simulink model "sampleModel1491"  (R2023a)
settings: Solver=VariableStepAuto  StartTime=0.0  StopTime=10.0  RelTol=1e-3
libraries: simulink x3, hdlsllib x2
settings Model: Creator=user1  LastModifiedBy=user1

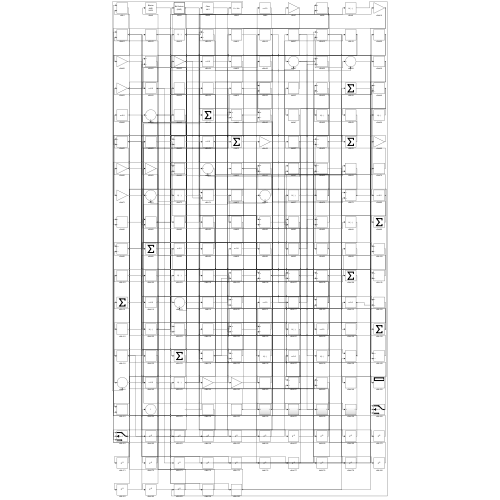
[thumbnail: Simulink's stored preview of the top-level diagram]
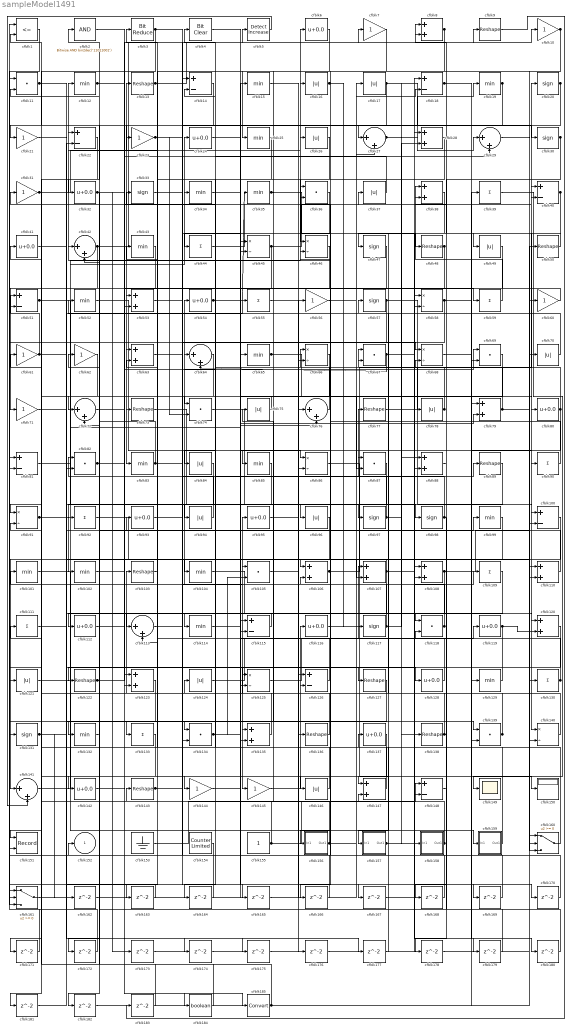
== system sampleModel1491 ==
  cfblk1 : RelationalOperator  Operator=<=  OutDataTypeStr=boolean  InputSameDT=off
  cfblk{7,10,21,23,31,56,60..62,71,144..145} (12 alike) : Gain
  cfblk{14,18,22,40,51,81,100,115,126,148} (10 alike) : Sum  Inputs=+-
  cfblk{12,15,19,25,34..35,43,52,65,83,85,99,101..102,104,114,129,132} (18 alike) : MinMax
  cfblk{9,13,48,50,73,77,89,103,122,127,136,138,143} (13 alike) : Reshape
  cfblk{11,36,67,69,74,82,87,105,118,134,139} (11 alike) : DotProduct  OutDataTypeStr=Inherit: Inherit via internal rule
  cfblk{8,28,38,53,63,79,88,106..108,110,120,123,135,147} (15 alike) : Sum
  cfblk{39,44,55,59,90,92,109,111,130,133} (10 alike) : Sum  Inputs=+
  cfblk{6,24,32,41,54,80,93,95,112,116,119,128,137,142} (14 alike) : Bias  Bias=0.0  SaturateOnIntegerOverflow=off
  cfblk{27,29,42,64,72,76,113,141} (8 alike) : Sum  Inputs=|++
  cfblk{20,30,33,47,57,97..98,117,131} (9 alike) : Signum
  cfblk{16..17,26,37,49,70,75,78,84,94,96,121,124,146} (14 alike) : Abs  SaturateOnIntegerOverflow=off
  cfblk{45..46,58,66,68,86,91,125,140} (9 alike) : Product  Inputs=*/  RndMeth=Zero  SaturateOnIntegerOverflow=on
  cfblk149 : Scope
  cfblk150 : Display
  cfblk151 : Record  FileSettingsInternal="{\"entries\":[{\"content\":{\"excelSettings\":{\"content\":{},\"type\":\"Streamout.ExcelSettings\"}},\"type\":\"Streamout.FileSettingStorage\",\"uuid\":\"\"}],\"packageUris\":[\"http:\\/\\/schema.mathworks.com\\/mf0\\/streamout_blocks\\/R2020a\"],\"version\":\"1.0\"}"  Layout=[1 1]  SignalsInternal="{\"entries\":[{\"content\":{\"signals\":[{\"content\":{\"blockPath\":[],\"dimensions\":[1],\"domain\":\"\",\"lineColor\":\"#a2142f\",\"plots\":[1],\"port\":1,\"signalID\":1220,\"signalName\":\"XY Graph:1\"},\"type\":\"RecordBlkView.Signal\",\"uuid\":\"\"},{\"content\":{\"blockPath\":[],\"dimensions\":[1],\"domain\":\"\",\"lineColor\":\"#139fff\",\"plots\":[1],\"port\":2,\"signalID\":1223,\"signalName\":\"XY Graph:2\"},\"type\":\"RecordBlkView.Signal\",\"uuid\":\"\"}]},\"type\":\"RecordBlkView.InputSignals\",\"uuid\":\"\"}],\"packageUris\":[\"http:\\/\\/schema.mathworks.com\\/mf0\\/streamout_blocks\\/R2020a\"],\"version\":\"1.0\"}"  VisualizationBindings="{\"xyplotplugin\":{\"info\":[{\"series\":[{\"bindingParametersList\":[{\"parameter\":\"X-Axis\",\"signalID\":1220,\"signalName\":\"XY Graph:1\"},{\"parameter\":\"Y-Axis\",\"signalID\":1223,\"signalName\":\"XY Graph:2\"}],\"seriesID\":24875}],\"subplotID\":1}]}}"  CompatibilityTag=XY  st=-1
  cfblk153 : Ground
  cfblk154 : hdlsllib/Sources/Counter Limited  uplimit=7  tsamp=-1
  cfblk155 : Constant  SampleTime=-1
  cfblk156 : Subsystem
      settings: LibrarySourceBlock=|
      | hdlsllib/Ports &
      | Subsystems/Subsystem
  cfblk157 : Subsystem
      settings: LibrarySourceBlock=|
      | hdlsllib/Ports &
      | Subsystems/Subsystem
  cfblk158 : Subsystem
      settings: LibrarySourceBlock=|
      | hdlsllib/Ports &
      | Subsystems/Subsystem
  cfblk159 : Subsystem
      settings: LibrarySourceBlock=|
      | hdlsllib/Ports &
      | Subsystems/Subsystem
  cfblk160 : Switch  SaturateOnIntegerOverflow=off  InputSameDT=off
  cfblk161 : Switch  SaturateOnIntegerOverflow=off  InputSameDT=off
  cfblk{162..183} (22 alike) : Delay  SampleTime=1
  cfblk184 : DataTypeConversion  OutDataTypeStr=boolean  SaturateOnIntegerOverflow=off  RndMeth=Floor
  cfblk185 : DataTypeConversion  SaturateOnIntegerOverflow=off  RndMeth=Floor
  cfblk2 : simulink/Logic and Bit Operations/Bitwise Operator  logicop=AND  UseBitMask=on  BitMask=bin2dec('11011001')  BitMaskRealWorld=Stored Integer
      settings: LibrarySourceBlock=|
      | hdlsllib/Logic and Bit
      | Operations/Bitwise
      | Operator
  cfblk3 : hdlsllib/Logic and Bit Operations/Bit Reduce  mode=AND
  cfblk4 : simulink/Logic and Bit Operations/Bit Clear  iBit=0
      settings: LibrarySourceBlock=|
      | hdlsllib/Logic and Bit
      | Operations/Bit Clear
  cfblk5 : simulink/Logic and Bit Operations/Detect Increase  vinit=0.0  OutDataTypeStr=boolean
      settings: LibrarySourceBlock=|
      | hdlsllib/Logic and Bit
      | Operations/Detect
      | Increase
  cfblk152 : Outport  VectorParamsAs1DForOutWhenUnconnected=off
  wires:
  cfblk42/1 -> cfblk10/1, cfblk127/1, cfblk82/2
  cfblk3/1 -> cfblk21/1, cfblk169/1
  cfblk126/1 -> cfblk12/1
  cfblk155/1 -> cfblk148/1, cfblk143/1
  cfblk90/1 -> cfblk42/1
  cfblk121/1 -> cfblk6/1
  cfblk128/1 -> cfblk22/1
  cfblk120/1 -> cfblk103/1
  cfblk39/1 -> cfblk149/1
  cfblk135/1 -> cfblk95/1
  cfblk67/1 -> cfblk64/2, cfblk179/1
  cfblk119/1 -> cfblk145/1, cfblk120/2
  cfblk12/1 -> cfblk59/1, cfblk184/1
  cfblk123/1 -> cfblk141/1
  cfblk127/1 -> cfblk133/1
  cfblk102/1 -> cfblk69/1
  cfblk14/1 -> cfblk83/1
  cfblk40/1 -> cfblk140/1, cfblk47/1
  cfblk144/1 -> cfblk119/1
  cfblk10/1 -> cfblk113/1, cfblk160/3
  cfblk117/1 -> cfblk54/1, cfblk88/1
  cfblk101/1 -> cfblk159/1(In1)
  cfblk54/1 -> cfblk35/1, cfblk84/1
  cfblk112/1 -> cfblk99/1
  cfblk8/1 -> cfblk25/1, cfblk36/1
  cfblk62/1 -> cfblk91/1
  cfblk5/1 -> cfblk141/2
  cfblk141/1 -> cfblk24/1
  cfblk76/1 -> cfblk31/1
  cfblk23/1 -> cfblk27/1, cfblk74/2
  cfblk78/1 -> cfblk67/1, cfblk67/2
  cfblk31/1 -> cfblk13/1, cfblk110/2
  cfblk59/1 -> cfblk38/1
  cfblk87/1 -> cfblk94/1
  cfblk57/1 -> cfblk100/1, cfblk151/2
  cfblk50/1 -> cfblk49/1
  cfblk48/1 -> cfblk147/1, cfblk88/2
  cfblk7/1 -> cfblk113/2
  cfblk51/1 -> cfblk96/1, cfblk175/1
  cfblk86/1 -> cfblk150/1
  cfblk73/1 -> cfblk115/1
  cfblk133/1 -> cfblk151/1
  cfblk116/1 -> cfblk148/2
  cfblk13/1 -> cfblk5/1, cfblk45/2
  cfblk60/1 -> cfblk53/1
  cfblk27/1 -> cfblk19/1, cfblk29/1, cfblk158/1(In1)
  cfblk49/1 -> cfblk71/1
  cfblk92/1 -> cfblk140/2
  cfblk29/1 -> cfblk110/1
  cfblk145/1 -> cfblk116/1
  cfblk160/1 -> cfblk61/1
  cfblk72/1 -> cfblk123/1
  cfblk147/1 -> cfblk34/1
  cfblk68/1 -> cfblk129/1
  cfblk66/1 -> cfblk144/1
  cfblk85/1 -> cfblk114/1
  cfblk53/1 -> cfblk68/1
  cfblk115/1 -> cfblk112/1
  cfblk139/1 -> cfblk57/1, cfblk124/1
  cfblk100/1 -> cfblk131/1
  cfblk106/1 -> cfblk20/1, cfblk18/2
  cfblk97/1 -> cfblk77/1, cfblk28/2
  cfblk80/1 -> cfblk52/1, cfblk135/2
  cfblk52/1 -> cfblk136/1
  cfblk161/1 -> cfblk17/1
  cfblk19/1 -> cfblk63/1, cfblk53/2
  cfblk91/1 -> cfblk15/1, cfblk97/1
  cfblk75/1 -> cfblk72/1
  cfblk4/1 -> cfblk80/1
  cfblk124/1 -> cfblk56/1
  cfblk36/1 -> cfblk44/1
  cfblk110/1 -> cfblk72/2
  cfblk159/1(Out1) -> cfblk64/1
  cfblk44/1 -> cfblk16/1
  cfblk96/1 -> cfblk142/1
  cfblk58/1 -> cfblk106/1, cfblk40/2
  cfblk125/1 -> cfblk69/2
  cfblk98/1 -> cfblk4/1, cfblk178/1
  cfblk93/1 -> cfblk128/1
  cfblk79/1 -> cfblk60/1, cfblk46/2
  cfblk65/1 -> cfblk126/1, cfblk87/2
  cfblk16/1 -> cfblk146/1, cfblk117/1
  cfblk45/1 -> cfblk37/1, cfblk51/2
  cfblk136/1 -> cfblk125/1
  cfblk2/1 -> cfblk185/1
  cfblk108/1 -> cfblk50/1, cfblk156/1(In1)
  cfblk63/1 -> cfblk7/1
  cfblk88/1 -> cfblk38/2
  cfblk129/1 -> cfblk122/1
  cfblk61/1 -> cfblk51/1, cfblk55/1
  cfblk77/1 -> cfblk39/1
  cfblk130/1 -> cfblk106/2, cfblk107/1
  cfblk74/1 -> cfblk98/1
  cfblk22/1 -> cfblk121/1
  cfblk114/1 -> cfblk79/2
  cfblk118/1 -> cfblk101/1, cfblk43/1
  cfblk20/1 -> cfblk32/1, cfblk66/2
  cfblk82/1 -> cfblk40/1, cfblk107/2
  cfblk21/1 -> cfblk134/1
  cfblk15/1 -> cfblk30/1
  cfblk28/1 -> cfblk46/1
  cfblk157/1(Out1) -> cfblk137/1, cfblk109/1
  cfblk17/1 -> cfblk81/2, cfblk130/1, cfblk138/1
  cfblk154/1 -> cfblk152/1
  cfblk107/1 -> cfblk78/1, cfblk104/1, cfblk115/2
  cfblk56/1 -> cfblk27/2
  cfblk84/1 -> cfblk134/2
  cfblk18/1 -> cfblk90/1, cfblk180/1
  cfblk26/1 -> cfblk73/1
  cfblk131/1 -> cfblk93/1, cfblk162/1
  cfblk105/1 -> cfblk89/1
  cfblk122/1 -> cfblk26/1, cfblk8/2
  cfblk30/1 -> cfblk48/1, cfblk160/2
  cfblk71/1 -> cfblk125/2
  cfblk89/1 -> cfblk102/1
  cfblk156/1(Out1) -> cfblk41/1, cfblk66/1, cfblk118/2
  cfblk104/1 -> cfblk118/1
  cfblk134/1 -> cfblk105/2, cfblk170/1
  cfblk24/1 -> cfblk86/1
  cfblk35/1 -> cfblk135/1, cfblk58/2
  cfblk95/1 -> cfblk108/2
  cfblk103/1 -> cfblk3/1
  cfblk140/1 -> cfblk111/1
  cfblk153/1 -> cfblk28/1
  cfblk11/1 -> cfblk139/1, cfblk120/1
  cfblk47/1 -> cfblk74/1
  cfblk38/1 -> cfblk157/1(In1)
  cfblk158/1(Out1) -> cfblk75/1, cfblk36/2
  cfblk83/1 -> cfblk11/2, cfblk9/1
  cfblk33/1 -> cfblk86/2
  cfblk46/1 -> cfblk92/1
  cfblk34/1 -> cfblk76/2
  cfblk37/1 -> cfblk14/2
  cfblk138/1 -> cfblk33/1, cfblk8/1
  cfblk81/1 -> cfblk65/1
  cfblk6/1 -> cfblk85/1
  cfblk94/1 -> cfblk82/1
  cfblk70/1 -> cfblk23/1
  cfblk43/1 -> cfblk123/2
  cfblk143/1 -> cfblk105/1, cfblk87/1
  cfblk32/1 -> cfblk132/1, cfblk29/2, cfblk173/1
  cfblk1/1 -> cfblk161/3
  cfblk146/1 -> cfblk63/2
  cfblk162/1 -> cfblk45/1
  cfblk99/1 -> cfblk163/1
  cfblk163/1 -> cfblk161/2
  cfblk25/1 -> cfblk164/1
  cfblk164/1 -> cfblk81/1
  cfblk113/1 -> cfblk165/1
  cfblk165/1 -> cfblk76/1
  cfblk69/1 -> cfblk166/1
  cfblk166/1 -> cfblk14/1
  cfblk41/1 -> cfblk167/1
  cfblk167/1 -> cfblk108/1
  cfblk148/1 -> cfblk168/1
  cfblk168/1 -> cfblk11/1
  cfblk169/1 -> cfblk1/2
  cfblk170/1 -> cfblk126/2
  cfblk64/1 -> cfblk171/1
  cfblk171/1 -> cfblk161/1
  cfblk132/1 -> cfblk172/1
  cfblk172/1 -> cfblk1/1
  cfblk173/1 -> cfblk139/2
  cfblk142/1 -> cfblk174/1
  cfblk174/1 -> cfblk18/1
  cfblk175/1 -> cfblk160/1
  cfblk55/1 -> cfblk176/1
  cfblk176/1 -> cfblk58/1
  cfblk111/1 -> cfblk177/1
  cfblk177/1 -> cfblk147/2
  cfblk178/1 -> cfblk100/2
  cfblk179/1 -> cfblk42/2
  cfblk180/1 -> cfblk68/2
  cfblk137/1 -> cfblk181/1
  cfblk181/1 -> cfblk22/2
  cfblk109/1 -> cfblk182/1
  cfblk182/1 -> cfblk79/1
  cfblk9/1 -> cfblk183/1
  cfblk183/1 -> cfblk91/2
  cfblk184/1 -> cfblk2/1
  cfblk185/1 -> cfblk70/1, cfblk62/1

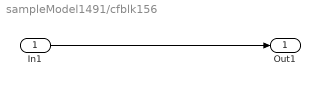
== system sampleModel1491/cfblk156 ==
  In1 : Inport
  Out1 : Outport
  wires:
  In1/1 -> Out1/1

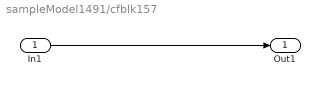
== system sampleModel1491/cfblk157 ==
  In1 : Inport
  Out1 : Outport
  wires:
  In1/1 -> Out1/1

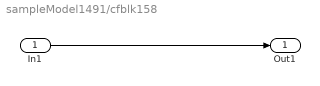
== system sampleModel1491/cfblk158 ==
  In1 : Inport
  Out1 : Outport
  wires:
  In1/1 -> Out1/1

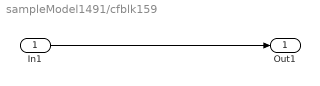
== system sampleModel1491/cfblk159 ==
  In1 : Inport
  Out1 : Outport
  wires:
  In1/1 -> Out1/1
